simulink model "oil_heater_model"  (R2020b)
settings: Solver=VariableStepAuto  StartTime=0.0  StopTime=2300  MaxStep=0.01  RelTol=1e-3
values from neighbouring files (symbols this model uses):
  A = 1    [oil_heater_starting_script.m]
  a_cv = interp1([353 383], a_cv_int, T_set, "linear", "extrap")    [oil_heater_starting_script.m]
  a_cx = interp1([353 383], a_cx_int, T_set, "linear", "extrap")    [oil_heater_starting_script.m]
  b_cv = interp1([353 383], b_cv_int, T_set, "linear", "extrap")    [oil_heater_starting_script.m]
  b_cx = interp1([353 383], b_cx_int, T_set, "linear", "extrap")    [oil_heater_starting_script.m]
  c_cv = interp1([353 383], c_cv_int, T_set, "linear", "extrap")    [oil_heater_starting_script.m]
  c_cx = interp1([353 383], c_cx_int, T_set, "linear", "extrap")    [oil_heater_starting_script.m]
  c_lookup = [1.962 2.049 2.137 2.4 2.619 2.838 3.058 3.277 3.452]    [oil_heater_starting_script.m]
  c_r = 0.4    [oil_heater_starting_script.m]
  d_lookup = [871 858 845 804 773 741 708 676 651]    [oil_heater_starting_script.m]
  m_r = 20    [oil_heater_starting_script.m]
  Q_tank = -7.4074e-06*(T_set-273-110)^4 - 8    (= -13.999994)    [oil_heater_starting_script.m]
  T1_i = T_set - 28    (= 325)    [oil_heater_starting_script.m]
  T2_i = T_set    (= 353)    [oil_heater_starting_script.m]
  T4_i = T_set - 13    (= 340)    [oil_heater_starting_script.m]
  T_lookup = [0 20 40 100 150 200 250 300 340] + 273    [oil_heater_starting_script.m]
  Tr_i = T_set    (= 353)    [oil_heater_starting_script.m]
  U = 0.27    [oil_heater_starting_script.m]
  v = 0.001278    [oil_heater_starting_script.m]
  v_e = 0.00384    [oil_heater_starting_script.m]
  v_h = 0.29    [oil_heater_starting_script.m]
  v_t = 0.167    [oil_heater_starting_script.m]
  W = 100    [oil_heater_starting_script.m]
settings Model: Creator=edizferit  LastModifiedBy=edizferit
settings SolverCC: AlgebraicLoopSolver=LineSearch

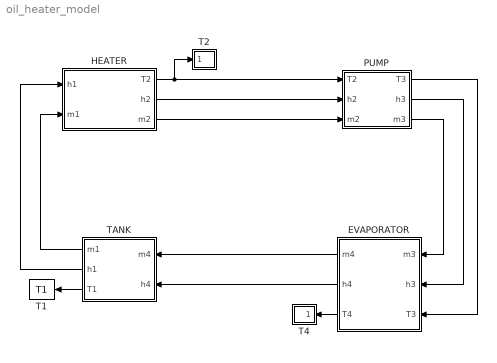
== system oil_heater_model ==
  EVAPORATOR : Subsystem
  HEATER : Subsystem
  PUMP : Subsystem
  T1 : ToWorkspace  VariableName=T1  SaveFormat=Timeseries  SampleTime=-1
  T2 : Subsystem
  T4 : Subsystem
  TANK : Subsystem
  wires:
  TANK/3(T1) -> T1/1
  TANK/1(m1) -> HEATER/2(m1)
  TANK/2(h1) -> HEATER/1(h1)
  HEATER/3(m2) -> PUMP/3(m2)
  HEATER/2(h2) -> PUMP/2(h2)
  EVAPORATOR/1(m4) -> TANK/1(m4)
  EVAPORATOR/2(h4) -> TANK/2(h4)
  PUMP/3(m3) -> EVAPORATOR/1(m3)
  PUMP/2(h3) -> EVAPORATOR/2(h3)
  EVAPORATOR/3(T4) -> T4/1(In1)
  HEATER/1(T2) -> PUMP/1(T2), T2/1(In1)
  PUMP/1(T3) -> EVAPORATOR/3(T3)

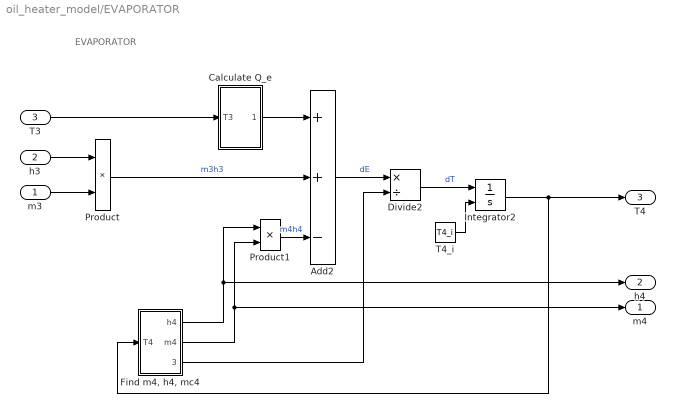
== system oil_heater_model/EVAPORATOR ==
  note: EVAPORATOR
  m3 : Inport
  h3 : Inport  Port=2
  T3 : Inport  Port=3
  Add2 : Sum  Inputs=++-
  Calculate Q_e : Subsystem
  Divide2 : Product  Inputs=*/
  "Find m4, h4, mc4" : Subsystem
  Integrator2 : Integrator  InitialConditionSource=external  InitialCondition=323
  Product : Product
  Product1 : Product
  T4_i : Constant  Value=T4_i
  m4 : Outport
  h4 : Outport  Port=2
  T4 : Outport  Port=3
  wires:
  "Find m4, h4, mc4"/1(h4) -> Product1/1, h4/1
  T4_i/1 -> Integrator2/2
  Add2/1 -> Divide2/1  "dE"
  "Find m4, h4, mc4"/3(mc4) -> Divide2/2
  "Find m4, h4, mc4"/2(m4) -> Product1/2, m4/1
  Integrator2/1 -> "Find m4, h4, mc4"/1(T4), T4/1
  Divide2/1 -> Integrator2/1  "dT"
  m3/1 -> Product/2
  h3/1 -> Product/1
  Product/1 -> Add2/2  "m3h3"
  Product1/1 -> Add2/3  "m4h4"
  Calculate Q_e/1(Q_e) -> Add2/1
  T3/1 -> Calculate Q_e/1(T3)

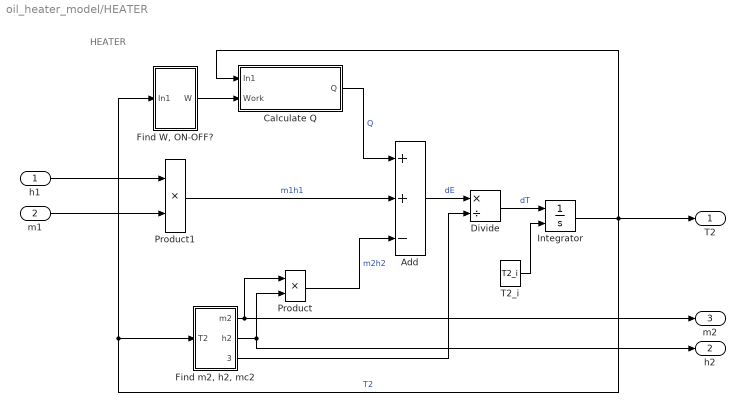
== system oil_heater_model/HEATER ==
  note: HEATER
  h1 : Inport
  m1 : Inport  Port=2
  Add : Sum  Inputs=++-
  Calculate Q : Subsystem
  Divide : Product  Inputs=*/
  "Find W, ON-OFF?" : Subsystem
  "Find m2, h2, mc2" : Subsystem
  Integrator : Integrator  InitialConditionSource=external  InitialCondition=323
  Product : Product
  Product1 : Product
  T2_i : Constant  Value=T2_i
  T2 : Outport
  h2 : Outport  Port=2
  m2 : Outport  Port=3
  wires:
  Integrator/1 -> "Find m2, h2, mc2"/1(T2), "Find W, ON-OFF?"/1(In1), T2/1, Calculate Q/1(In1)  "T2"
  Add/1 -> Divide/1  "dE"
  "Find m2, h2, mc2"/3(mc2) -> Divide/2
  Calculate Q/1(Q) -> Add/1  "Q"
  T2_i/1 -> Integrator/2
  "Find m2, h2, mc2"/2(h2) -> h2/1, Product/2
  "Find m2, h2, mc2"/1(m2) -> m2/1, Product/1
  "Find W, ON-OFF?"/1(W) -> Calculate Q/2(Work)
  Divide/1 -> Integrator/1  "dT"
  Product/1 -> Add/3  "m2h2"
  h1/1 -> Product1/1
  m1/1 -> Product1/2
  Product1/1 -> Add/2  "m1h1"

== system oil_heater_model/PUMP ==
  T2 : Inport
  h2 : Inport  Port=2
  m2 : Inport  Port=3
  T3 : Outport
  h3 : Outport  Port=2
  m3 : Outport  Port=3
  wires:
  m2/1 -> m3/1
  h2/1 -> h3/1
  T2/1 -> T3/1

== system oil_heater_model/T2 ==
  In1 : Inport
  Time Step - H : Subsystem
  To Workspace3 : ToWorkspace  VariableName=T2_step  SaveFormat=Timeseries  SampleTime=-1
  To Workspace4 : ToWorkspace  VariableName=T2  SaveFormat=Timeseries  SampleTime=-1
  wires:
  In1/1 -> To Workspace4/1, Time Step - H/1(T2)
  Time Step - H/1(Out1) -> To Workspace3/1

== system oil_heater_model/T4 ==
  In1 : Inport
  Time Step - E : Subsystem
  To Workspace1 : ToWorkspace  VariableName=T4  SaveFormat=Timeseries  SampleTime=-1
  To Workspace5 : ToWorkspace  VariableName=T4_step  SaveFormat=Timeseries  SampleTime=-1
  wires:
  In1/1 -> Time Step - E/1(T4), To Workspace1/1
  Time Step - E/1(Out1) -> To Workspace5/1

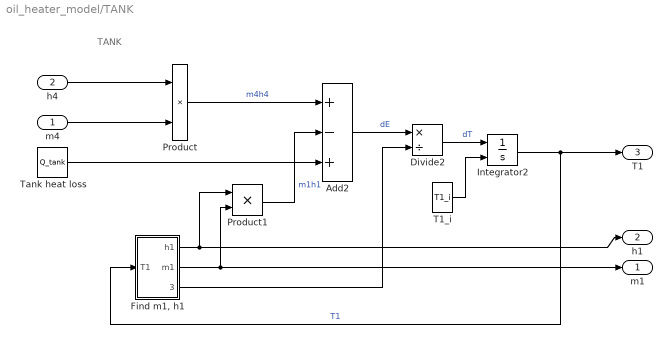
== system oil_heater_model/TANK ==
  note: TANK
  m4 : Inport
  h4 : Inport  Port=2
  Add2 : Sum  Inputs=+-+
  Divide2 : Product  Inputs=*/
  "Find m1, h1" : Subsystem
  Integrator2 : Integrator  InitialConditionSource=external  InitialCondition=323
  Product : Product
  Product1 : Product
  T1_i : Constant  Value=T1_i
  Tank heat loss : Constant  Value=Q_tank
  m1 : Outport
  h1 : Outport  Port=2
  T1 : Outport  Port=3
  wires:
  T1_i/1 -> Integrator2/2
  Integrator2/1 -> "Find m1, h1"/1(T1), T1/1  "T1"
  "Find m1, h1"/1(h1) -> Product1/1, h1/1
  "Find m1, h1"/2(m1) -> m1/1, Product1/2
  "Find m1, h1"/3(mc1) -> Divide2/2
  Divide2/1 -> Integrator2/1  "dT"
  Add2/1 -> Divide2/1  "dE"
  Product/1 -> Add2/1  "m4h4"
  h4/1 -> Product/1
  m4/1 -> Product/2
  Product1/1 -> Add2/2  "m1h1"
  Tank heat loss/1 -> Add2/3

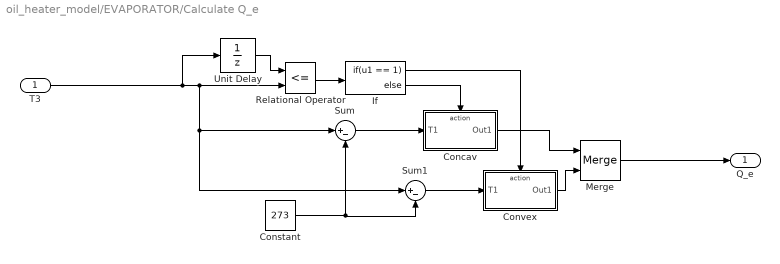
== system oil_heater_model/EVAPORATOR/Calculate Q_e ==
  T3 : Inport
  Concav : Subsystem  TreatAsAtomicUnit=on
  Constant : Constant  Value=273
  Convex : Subsystem  TreatAsAtomicUnit=on
  If : If  IfExpression=u1 == 1
  Merge : Merge
  Relational Operator : RelationalOperator  Operator=<=  OutDataTypeStr=boolean  RndMeth=Simplest
  Sum : Sum  Inputs=|+-
  Sum1 : Sum  Inputs=|+-
  Unit Delay : UnitDelay  SampleTime=-1  HasFrameUpgradeWarning=on
  Q_e : Outport
  wires:
  Relational Operator/1 -> If/1
  Unit Delay/1 -> Relational Operator/1
  T3/1 -> Sum1/1, Sum/1, Relational Operator/2, Unit Delay/1
  Concav/1(Out1) -> Merge/1
  If/1 -> Convex/Action
  If/2 -> Concav/Action
  Merge/1 -> Q_e/1
  Sum/1 -> Concav/1(T1)
  Sum1/1 -> Convex/1(T1)
  Constant/1 -> Sum1/2, Sum/2
  Convex/1(Out1) -> Merge/2

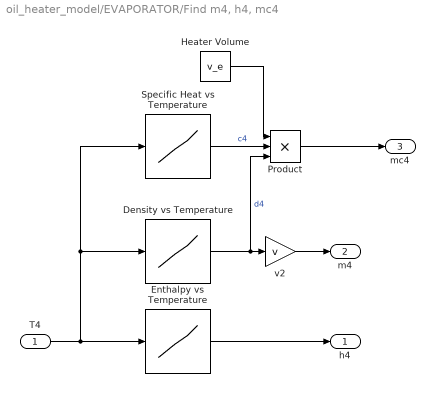
== system oil_heater_model/EVAPORATOR/Find m4, h4, mc4 ==
  T4 : Inport
  Density vs Temperature : Lookup_n-D  NumberOfTableDimensions=1  BreakpointsForDimension1=T_lookup  UseOneInputPortForAllInputData=on  Table=d_lookup  InternalRulePriority=Speed  RndMeth=Simplest  InputSameDT=on
  Enthalpy vs Temperature : Lookup_n-D  NumberOfTableDimensions=1  BreakpointsForDimension1=[273:373]  UseOneInputPortForAllInputData=on  Table=[560:2:760, ]  InternalRulePriority=Speed  RndMeth=Simplest  InputSameDT=on
  Heater Volume : Constant  Value=v_e
  Product : Product  Inputs=3
  Specific Heat vs Temperature : Lookup_n-D  NumberOfTableDimensions=1  BreakpointsForDimension1=T_lookup  UseOneInputPortForAllInputData=on  Table=c_lookup  InternalRulePriority=Speed  RndMeth=Simplest  InputSameDT=on
  v2 : Gain  Gain=v
  h4 : Outport
  m4 : Outport  Port=2
  mc4 : Outport  Port=3
  wires:
  v2/1 -> m4/1
  Enthalpy vs Temperature/1 -> h4/1
  Product/1 -> mc4/1
  T4/1 -> Enthalpy vs Temperature/1, Specific Heat vs Temperature/1, Density vs Temperature/1
  Heater Volume/1 -> Product/1
  Specific Heat vs Temperature/1 -> Product/2  "c4"
  Density vs Temperature/1 -> Product/3, v2/1  "d4"

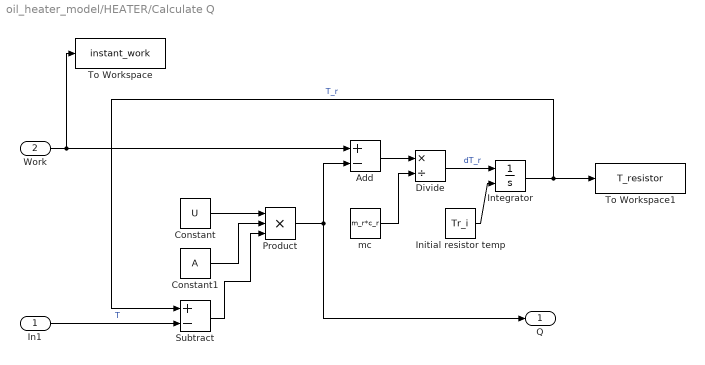
== system oil_heater_model/HEATER/Calculate Q ==
  In1 : Inport
  Work : Inport  Port=2
  Add : Sum  Inputs=+-
  Constant : Constant  Value=U
  Constant1 : Constant  Value=A
  Divide : Product  Inputs=*/
  Initial resistor temp : Constant  Value=Tr_i
  Integrator : Integrator  InitialConditionSource=external  InitialCondition=293
  Product : Product  Inputs=3
  Subtract : Sum  Inputs=+-
  To Workspace : ToWorkspace  VariableName=instant_work  SaveFormat=Timeseries  SampleTime=-1
  To Workspace1 : ToWorkspace  VariableName=T_resistor  SaveFormat=Timeseries  SampleTime=-1
  mc : Constant  Value=m_r*c_r
  Q : Outport
  wires:
  Work/1 -> To Workspace/1, Add/1
  Product/1 -> Q/1, Add/2
  Constant/1 -> Product/1
  Constant1/1 -> Product/2
  In1/1 -> Subtract/2  "T"
  Subtract/1 -> Product/3
  Integrator/1 -> Subtract/1, To Workspace1/1  "T_r"
  Add/1 -> Divide/1
  Divide/1 -> Integrator/1  "dT_r"
  mc/1 -> Divide/2
  Initial resistor temp/1 -> Integrator/2

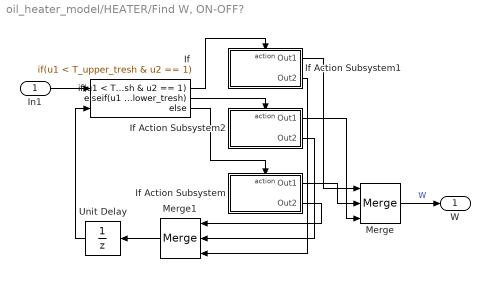
== system oil_heater_model/HEATER/Find W, ON-OFF? ==
  In1 : Inport
  If : If  NumInputs=2  IfExpression=u1 < T_upper_tresh & u2 == 1  ElseIfExpressions=u1 < T_lower_tresh  ZeroCross=off
  If Action Subsystem : Subsystem  TreatAsAtomicUnit=on
  If Action Subsystem1 : Subsystem  TreatAsAtomicUnit=on
  If Action Subsystem2 : Subsystem  TreatAsAtomicUnit=on
  Merge : Merge  Inputs=3
  Merge1 : Merge  Inputs=3  InitialOutput=[1]
  Unit Delay : UnitDelay  SampleTime=-1  HasFrameUpgradeWarning=on
  W : Outport
  wires:
  If/2 -> If Action Subsystem2/Action
  If/1 -> If Action Subsystem1/Action
  If Action Subsystem2/1(Out1) -> Merge/3
  If Action Subsystem1/2(Out2) -> Merge1/3
  Unit Delay/1 -> If/2
  If Action Subsystem2/2(Out2) -> Merge1/2
  If Action Subsystem1/1(Out1) -> Merge/1
  If/3 -> If Action Subsystem/Action
  If Action Subsystem/2(Out2) -> Merge1/1
  Merge1/1 -> Unit Delay/1
  If Action Subsystem/1(Out1) -> Merge/2
  In1/1 -> If/1
  Merge/1 -> W/1  "W"

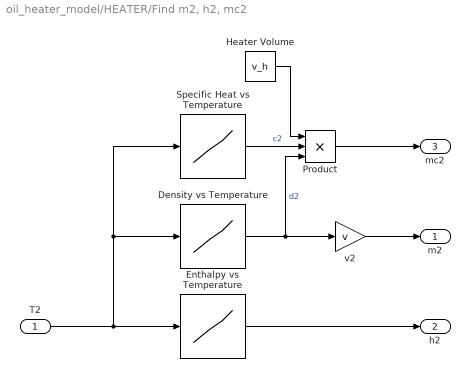
== system oil_heater_model/HEATER/Find m2, h2, mc2 ==
  T2 : Inport
  Density vs Temperature : Lookup_n-D  NumberOfTableDimensions=1  BreakpointsForDimension1=T_lookup  UseOneInputPortForAllInputData=on  Table=d_lookup  InternalRulePriority=Speed  RndMeth=Simplest  InputSameDT=on
  Enthalpy vs Temperature : Lookup_n-D  NumberOfTableDimensions=1  BreakpointsForDimension1=[273:373]  Table=[560:2:760, ]  InternalRulePriority=Speed  RndMeth=Simplest  InputSameDT=on
  Heater Volume : Constant  Value=v_h
  Product : Product  Inputs=3
  Specific Heat vs Temperature : Lookup_n-D  NumberOfTableDimensions=1  BreakpointsForDimension1=T_lookup  UseOneInputPortForAllInputData=on  Table=c_lookup  InternalRulePriority=Speed  RndMeth=Simplest  InputSameDT=on
  v2 : Gain  Gain=v
  m2 : Outport
  h2 : Outport  Port=2
  mc2 : Outport  Port=3
  wires:
  T2/1 -> Specific Heat vs Temperature/1, Density vs Temperature/1, Enthalpy vs Temperature/1
  Density vs Temperature/1 -> Product/3, v2/1  "d2"
  Enthalpy vs Temperature/1 -> h2/1
  v2/1 -> m2/1
  Specific Heat vs Temperature/1 -> Product/2  "c2"
  Heater Volume/1 -> Product/1
  Product/1 -> mc2/1

== system oil_heater_model/T2/Time Step - H ==
  T2 : Inport
  Pulse Generator : DiscretePulseGenerator  PulseType=Time based  Period=1
  Triggered Subsystem : Subsystem  TreatAsAtomicUnit=on
  Out1 : Outport
  wires:
  Triggered Subsystem/1(Out1) -> Out1/1
  Pulse Generator/1 -> Triggered Subsystem/Enable, Triggered Subsystem/Trigger
  T2/1 -> Triggered Subsystem/1(T2)

== system oil_heater_model/T4/Time Step - E ==
  T4 : Inport
  Pulse Generator : DiscretePulseGenerator  PulseType=Time based  Period=1
  Triggered Subsystem : Subsystem  TreatAsAtomicUnit=on
  Out1 : Outport
  wires:
  Pulse Generator/1 -> Triggered Subsystem/Enable, Triggered Subsystem/Trigger
  T4/1 -> Triggered Subsystem/1(T4)
  Triggered Subsystem/1(Out1) -> Out1/1

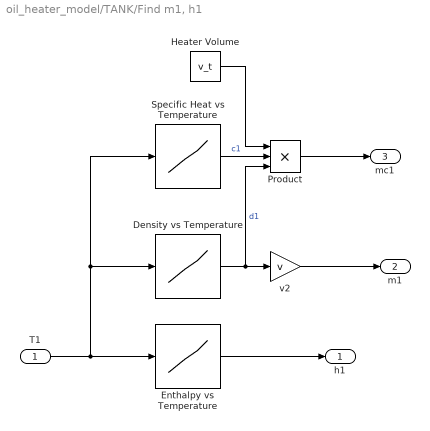
== system oil_heater_model/TANK/Find m1, h1 ==
  T1 : Inport
  Density vs Temperature : Lookup_n-D  NumberOfTableDimensions=1  BreakpointsForDimension1=T_lookup  UseOneInputPortForAllInputData=on  Table=d_lookup  InternalRulePriority=Speed  RndMeth=Simplest  InputSameDT=on
  Enthalpy vs Temperature : Lookup_n-D  NumberOfTableDimensions=1  BreakpointsForDimension1=[273:373]  UseOneInputPortForAllInputData=on  Table=[560:2:760, ]  InternalRulePriority=Speed  RndMeth=Simplest  InputSameDT=on
  Heater Volume : Constant  Value=v_t
  Product : Product  Inputs=3
  Specific Heat vs Temperature : Lookup_n-D  NumberOfTableDimensions=1  BreakpointsForDimension1=T_lookup  UseOneInputPortForAllInputData=on  Table=c_lookup  InternalRulePriority=Speed  RndMeth=Simplest  InputSameDT=on
  v2 : Gain  Gain=v
  h1 : Outport
  m1 : Outport  Port=2
  mc1 : Outport  Port=3
  wires:
  Enthalpy vs Temperature/1 -> h1/1
  v2/1 -> m1/1
  Product/1 -> mc1/1
  T1/1 -> Enthalpy vs Temperature/1, Specific Heat vs Temperature/1, Density vs Temperature/1
  Heater Volume/1 -> Product/1
  Specific Heat vs Temperature/1 -> Product/2  "c1"
  Density vs Temperature/1 -> Product/3, v2/1  "d1"

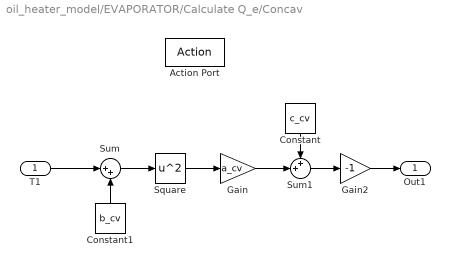
== system oil_heater_model/EVAPORATOR/Calculate Q_e/Concav ==
  T1 : Inport
  Action Port : ActionPort  ActionPortLabel=else
  Constant : Constant  Value=c_cv
  Constant1 : Constant  Value=b_cv
  Gain : Gain  Gain=a_cv
  Gain2 : Gain  Gain=-1
  Square : Math  Operator=square  SaturateOnIntegerOverflow=on
  Sum : Sum  Inputs=|++
  Sum1 : Sum  Inputs=++|
  Out1 : Outport
  wires:
  Sum1/1 -> Gain2/1
  Gain2/1 -> Out1/1
  Square/1 -> Gain/1
  Sum/1 -> Square/1
  T1/1 -> Sum/1
  Constant1/1 -> Sum/2
  Gain/1 -> Sum1/2
  Constant/1 -> Sum1/1

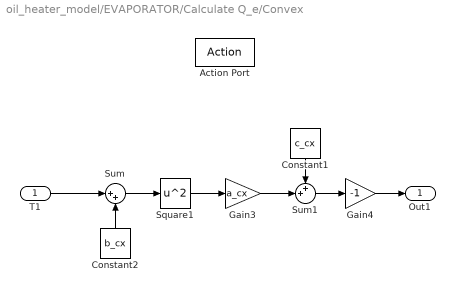
== system oil_heater_model/EVAPORATOR/Calculate Q_e/Convex ==
  T1 : Inport
  Action Port : ActionPort  ActionPortLabel=if(u1 == 1)
  Constant1 : Constant  Value=c_cx
  Constant2 : Constant  Value=b_cx
  Gain3 : Gain  Gain=a_cx
  Gain4 : Gain  Gain=-1
  Square1 : Math  Operator=square  SaturateOnIntegerOverflow=on
  Sum : Sum  Inputs=|++
  Sum1 : Sum  Inputs=++|
  Out1 : Outport
  wires:
  Gain4/1 -> Out1/1
  T1/1 -> Sum/1
  Sum1/1 -> Gain4/1
  Sum/1 -> Square1/1
  Constant2/1 -> Sum/2
  Constant1/1 -> Sum1/1
  Square1/1 -> Gain3/1
  Gain3/1 -> Sum1/2

== system oil_heater_model/HEATER/Find W, ON-OFF?/If Action Subsystem ==
  Action Port : ActionPort  ActionPortLabel=else
  Constant1 : Constant
  Constant2 : Constant  Value=0
  Gain : Gain  Gain=-1
  Out1 : Outport
  Out2 : Outport  Port=2  InitialOutput=[1]
  wires:
  Gain/1 -> Out2/1
  Constant1/1 -> Gain/1
  Constant2/1 -> Out1/1

== system oil_heater_model/HEATER/Find W, ON-OFF?/If Action Subsystem1 ==
  Action Port : ActionPort  ActionPortLabel=if(u1 < T_upper_tresh & u2 == 1)
  Constant1 : Constant
  Constant2 : Constant  Value=W
  Out1 : Outport
  Out2 : Outport  Port=2  InitialOutput=[1]
  wires:
  Constant1/1 -> Out2/1
  Constant2/1 -> Out1/1

== system oil_heater_model/HEATER/Find W, ON-OFF?/If Action Subsystem2 ==
  Action Port : ActionPort  ActionPortLabel=elseif(u1 < T_lower_tresh)
  Constant1 : Constant
  Constant2 : Constant  Value=W
  Out1 : Outport
  Out2 : Outport  Port=2  InitialOutput=[1]
  wires:
  Constant1/1 -> Out2/1
  Constant2/1 -> Out1/1

== system oil_heater_model/T2/Time Step - H/Triggered Subsystem ==
  T2 : Inport
  Enable : EnablePort  StatesWhenEnabling=reset
  Trigger : TriggerPort  VariantControl=Variant
  Out1 : Outport  OutputWhenDisabled=reset  InitialOutput=0
  wires:
  T2/1 -> Out1/1

== system oil_heater_model/T4/Time Step - E/Triggered Subsystem ==
  T4 : Inport
  Enable : EnablePort  StatesWhenEnabling=reset
  Trigger : TriggerPort  VariantControl=Variant
  Out1 : Outport  OutputWhenDisabled=reset  InitialOutput=0
  wires:
  T4/1 -> Out1/1
